simulink model "ExistingMIMOmodeling"  (R2020a)
settings: Solver=VariableStepAuto  StartTime=0.0  StopTime=150000  RelTol=1e-3
undefined symbols (not defined in the file): R1Kd, R2Kd, R3Kd
libraries: cstblocks x6
settings Model: Creator=User  LastModifiedBy=User
settings SolverCC: AlgebraicLoopSolver=LineSearch

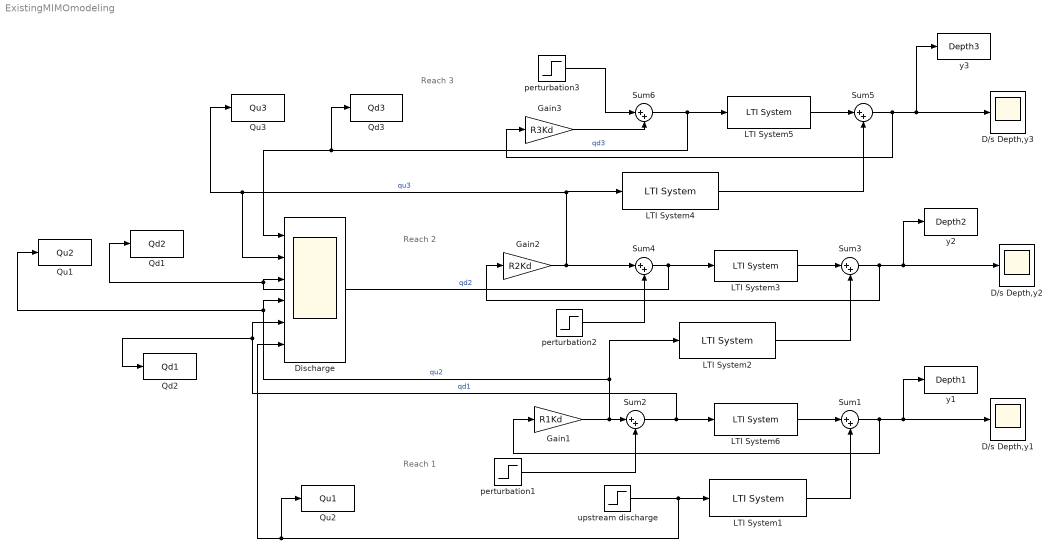
== system ExistingMIMOmodeling ==
  note: Reach 1
  note: Reach 2
  note: Reach 3
  D/s Depth,y1 : Scope
  D/s Depth,y2 : Scope
  D/s Depth,y3 : Scope
  Discharge : Scope  NumInputPorts=6
  Gain1 : Gain  Gain=R1Kd
  Gain2 : Gain  Gain=R2Kd
  Gain3 : Gain  Gain=R3Kd
  LTI System1 : cstblocks/LTI System  sys=R1P21  IC=[]
  LTI System2 : cstblocks/LTI System  sys=R2P21  IC=[]
  LTI System3 : cstblocks/LTI System  sys=R2P22  IC=[]
  LTI System4 : cstblocks/LTI System  sys=R3P21  IC=[]
  LTI System5 : cstblocks/LTI System  sys=R3P22  IC=[]
  LTI System6 : cstblocks/LTI System  sys=R1P22  IC=[]
  Qd1 : ToWorkspace  VariableName=Qd2  SaveFormat=Timeseries  SampleTime=-1
  Qd2 : ToWorkspace  VariableName=Qd1  SaveFormat=Timeseries  SampleTime=-1
  Qd3 : ToWorkspace  VariableName=Qd3  SaveFormat=Timeseries  SampleTime=-1
  Qu1 : ToWorkspace  VariableName=Qu2  SaveFormat=Timeseries  SampleTime=-1
  Qu2 : ToWorkspace  VariableName=Qu1  SaveFormat=Timeseries  SampleTime=-1
  Qu3 : ToWorkspace  VariableName=Qu3  SaveFormat=Timeseries  SampleTime=-1
  Sum{1..6} (6 alike) : Sum  Inputs=|++
  perturbation1 : Step  Time=1200  After=0  SampleTime=0
  perturbation2 : Step  Time=1200  After=0.15  SampleTime=0
  perturbation3 : Step  Time=1200  After=0  SampleTime=0
  upstream discharge : Step  Time=1200  After=0  SampleTime=0
  y1 : ToWorkspace  VariableName=Depth1  SaveFormat=Timeseries  SampleTime=-1
  y2 : ToWorkspace  VariableName=Depth2  SaveFormat=Timeseries  SampleTime=-1
  y3 : ToWorkspace  VariableName=Depth3  SaveFormat=Timeseries  SampleTime=-1
  wires:
  LTI System3/1 -> Sum3/1
  Sum3/1 -> Gain2/1, D/s Depth,y2/1, y2/1
  Sum2/1 -> Qd2/1, Discharge/5, LTI System6/1  "qd1"
  LTI System2/1 -> Sum3/2
  LTI System5/1 -> Sum5/1
  perturbation3/1 -> Sum6/1
  Sum6/1 -> Discharge/1, Qd3/1, LTI System5/1  "qd3"
  Sum5/1 -> Gain3/1, D/s Depth,y3/1, y3/1
  Gain3/1 -> Sum6/2
  LTI System4/1 -> Sum5/2
  LTI System1/1 -> Sum1/2
  upstream discharge/1 -> Qu2/1, Discharge/6, LTI System1/1
  Sum1/1 -> Gain1/1, D/s Depth,y1/1, y1/1
  LTI System6/1 -> Sum1/1
  Gain2/1 -> Qu3/1, Discharge/2, LTI System4/1, Sum4/1  "qu3"
  perturbation2/1 -> Sum4/2
  Sum4/1 -> Qd1/1, Discharge/3, LTI System3/1  "qd2"
  Gain1/1 -> Qu1/1, Discharge/4, LTI System2/1, Sum2/1  "qu2"
  perturbation1/1 -> Sum2/2
